simulink model "thhtt_lab3"  (R2018b)
settings: Solver=VariableStepAuto  StartTime=0.0  StopTime=10.0  RelTol=1e-3
libraries: dsparch4 x1, commsynccomp2 x1, dspsigops x1
settings Model: Creator=PC  LastModifiedBy=PC

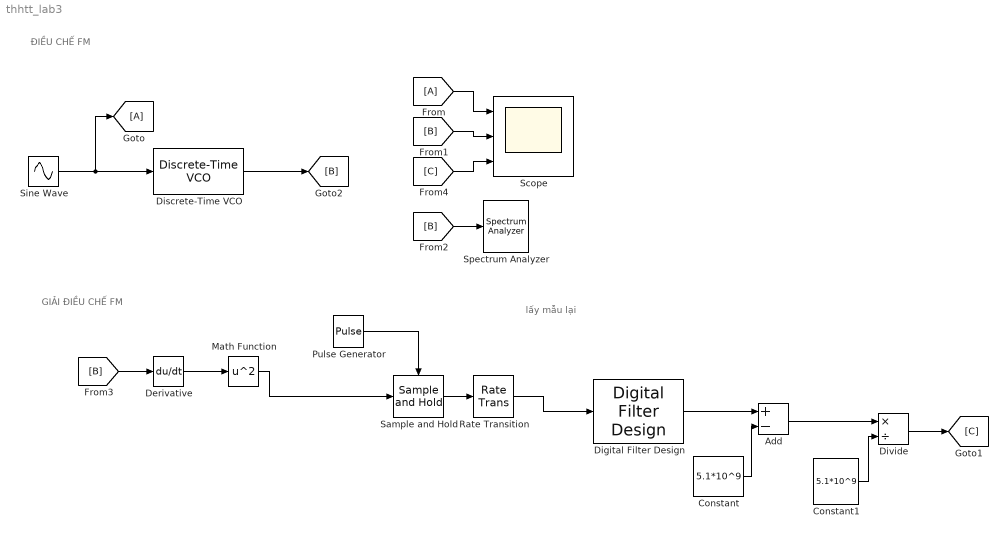
== system thhtt_lab3 ==
  note: ĐIỀU CHẾ FM
  note: GIẢI ĐIỀU CHẾ FM
  note: lấy mẫu lại
  Add : Sum  Inputs=+-
  Constant : Constant  Value=5.1*10^9  VectorParams1D=off
  Constant1 : Constant  Value=5.1*10^9
  Derivative : Derivative
  Digital Filter Design : dsparch4/Digital Filter Design  mwdsp_browser_bugfix_var=off
  Discrete-Time VCO : commsynccomp2/Discrete-Time VCO  Ac=5  Fc=3000  Kc=2000  Ph=0  ts=1/20000
      settings: SourceProductName=Communications System Toolbox  SourceProductBaseCode=CM
  Divide : Product  Inputs=*/
  Math Function : Math  Operator=square  SaturateOnIntegerOverflow=on
  Pulse Generator : DiscretePulseGenerator  PulseType=Time based  Period=1/20000  PulseWidth=5
  Rate Transition : RateTransition
  Sample and Hold : dspsigops/Sample and Hold  trig=Rising edge  initCond=0  latchinput=off
  Scope : Scope  NumInputPorts=3
  Sine Wave : Sin  Frequency=2*pi*500  SampleTime=1/20000
  Spectrum Analyzer : SpectrumAnalyzer
  wires:
  Discrete-Time VCO/1 -> [B]
  Sine Wave/1 -> [A], Discrete-Time VCO/1
  [A] -> Scope/1
  [B] -> Scope/2
  [B] -> Spectrum Analyzer/1
  [B] -> Derivative/1
  Derivative/1 -> Math Function/1
  Pulse Generator/1 -> Sample and Hold/Trigger
  Math Function/1 -> Sample and Hold/1
  Sample and Hold/1 -> Rate Transition/1
  Rate Transition/1 -> Digital Filter Design/1
  Digital Filter Design/1 -> Add/1
  Constant/1 -> Add/2
  [C] -> Scope/3
  Add/1 -> Divide/1
  Divide/1 -> [C]
  Constant1/1 -> Divide/2
